simulink model "untitled"  (R2019b)
settings: Solver=FixedStepAuto  StartTime=0.0  StopTime=10.0  FixedStep=0.001  RelTol=1e-3
settings Model: Creator=y0n  LastModifiedBy=y0n

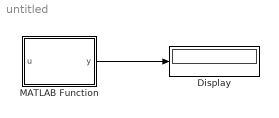
== system untitled ==
  Display : Display
  MATLAB Function : MATLAB Function  TreatAsAtomicUnit=on
  wires:
  MATLAB Function/1(y) -> Display/1

== matlab function untitled/MATLAB Function ==
  data: u input; y output
function y = fcn(u)

y = string(char([54 51 48]));
